simulink library "beamform"  (Simulink 7.0)
libraries: xbsIndex_r4 x216, beamform x73
(part 1 of 2)
settings Model: Creator=Administrator  LastModifiedBy=Administrator

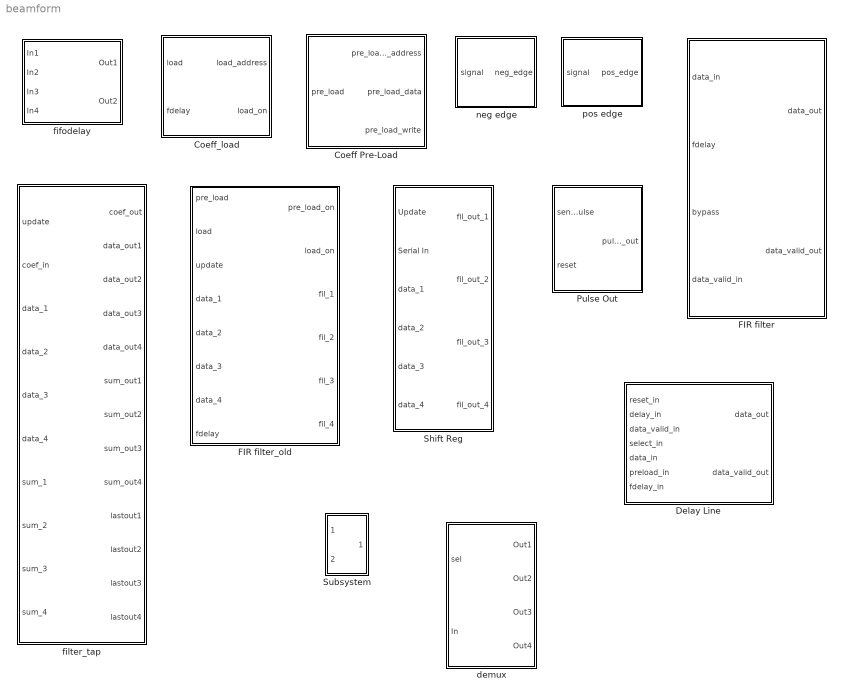
== system beamform ==
  Coeff Pre-Load : Subsystem  mask{N=20, T=10, bin_pnt=6, file='cfile.mat'}
      mask prompts: N "No of Filters"; T "No of Taps"; bin_pnt "Binary Point"; file "Coefficients File"
      mask init:
      | load(file)
  Coeff_load : Subsystem  mask{nfilters=10, ntaps=20}
      mask prompts: nfilters "Number of FD filters"; ntaps "Number of Taps per filter"
      mask init:
      | coef_load;
  Delay Line : Subsystem
  FIR filter : Subsystem
  FIR filter_old : Subsystem  mask{ntaps=4, nfilters=4, cfile=test.mat, bin_pnt=6}
      mask prompts: ntaps "No of Taps"; nfilters "No of Filters"; cfile "Coefficients"; bin_pnt "Binary Point"
      mask init:
      | load(cfile);
  Pulse Out : Subsystem
  Shift Reg : Subsystem  mask{n=20, bin_point=6}
      mask prompts: n "No of taps"; bin_point "Binary Point"
      mask init:
      | shift_reg;
  Subsystem : Subsystem
  demux : Subsystem  mask{n_bits=20}
  fifodelay : Subsystem  mask{depth=1}
      mask init:
      | drawfifo;
      mask Display:
      | port_label('input',1,'reset');
      | port_label('input',2,'data_in');
      | port_label('input',3,'delay');
      | port_label('input',4,'data_valid');
      | port_label('output',1,'data_out');
      | port_label('output',2,'data_valid');
  filter_tap : Subsystem  mask{n_bits=8, bnpnt=6, mux_latency=0, add_latency=2, mult_latency=3, qn_bits=18, qbnpnt=16}
      mask prompts: n_bits "Coefficient bit width"; bnpnt "Coeff & Data Binary Point"; mux_latency "Multiplexer Latency"; add_latency "Add Latency"; mult_latency "Multiplier Latency"; qn_bits "Quiscent Bitwdith"; qbnpnt "Quiscent Binary Point"
  neg edge : Subsystem  mask{add_latency=1}
  pos edge : Subsystem  mask{add_latency=1}

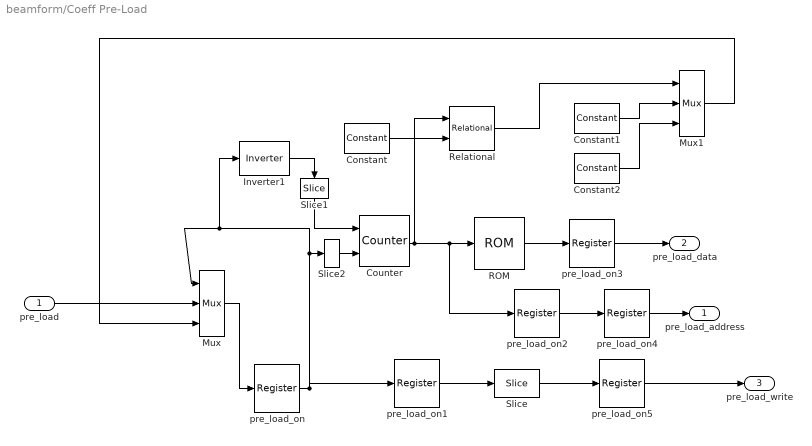
== system beamform/Coeff Pre-Load ==
  pre_load : Inport  OutDataType=sfix(16)  OutScaling=2^0
  Constant : xbsIndex_r4/Constant  arith_type=Unsigned  const=N*T-1  n_bits=ceil(log2(N*T-1))  bin_pt=0  explicit_period=on  period=1  equ=P=C  opselect=C  inp2=PCIN>>17  opr=+  inp1=P  carry=CIN  dbl_ovrd=off  block_type=constant
  Constant1 : xbsIndex_r4/Constant  arith_type=Unsigned  const=1  n_bits=1  bin_pt=0  explicit_period=on  period=1  equ=P=C  opselect=C  inp2=PCIN>>17  opr=+  inp1=P  carry=CIN  dbl_ovrd=off  block_type=constant
  Constant2 : xbsIndex_r4/Constant  arith_type=Unsigned  const=0  n_bits=1  bin_pt=0  explicit_period=on  period=1  equ=P=C  opselect=C  inp2=PCIN>>17  opr=+  inp1=P  carry=CIN  dbl_ovrd=off  block_type=constant
  Counter : xbsIndex_r4/Counter  cnt_type=Count Limited  cnt_to=N*T-1  operation=Up  start_count=0  cnt_by_val=1  arith_type=Unsigned  n_bits=ceil(log2(N*T))  bin_pt=0  load_pin=off  rst=on  en=on  explicit_period=off  period=1  dbl_ovrd=off  use_behavioral_HDL=off  use_rpm=on  implementation=Fabric  block_type=counter
      settings: xl_area=[0, 0, 0, 0, 0, 0, 0]
  Inverter1 : xbsIndex_r4/Inverter  en=off  latency=0  dbl_ovrd=off  block_type=inv
      settings: xl_area=[0, 0, 0, 0, 0, 0, 0]
  Mux : xbsIndex_r4/Mux  inputs=2  en=off  latency=0  precision=Full  arith_type=Unsigned  n_bits=1  bin_pt=0  quantization=Truncate  overflow=Wrap  dbl_ovrd=off  block_type=mux
      settings: xl_area=[0, 0, 0, 0, 0, 0, 0]
  Mux1 : xbsIndex_r4/Mux  inputs=2  en=off  latency=0  precision=Full  arith_type=Unsigned  n_bits=1  bin_pt=0  quantization=Truncate  overflow=Wrap  dbl_ovrd=off  block_type=mux
      settings: xl_area=[0, 0, 0, 0, 0, 0, 0]
  ROM : xbsIndex_r4/ROM  depth=N*T  initVector=A  distributed_mem=Block RAM  rst=off  init_reg=0  en=off  latency=1  arith_type="Signed  (2's comp)"  n_bits=18  bin_pt=16  dbl_ovrd=off  optimize=Area  use_rpm=off  block_type=sprom
      settings: xl_area=[0, 0, 0, 0, 0, 0, 0]  block_version=10.1.3
  Relational : xbsIndex_r4/Relational  mode=a>=b  en=off  latency=1  dbl_ovrd=off  block_type=relational
      settings: xl_area=[0, 0, 0, 0, 0, 0, 0]  block_version=10.1.3
  Slice : xbsIndex_r4/Slice  nbits=1  boolean_output=on  mode=Upper Bit Location + Width  bit1=0  base1=MSB of Input  bit0=0  base0=LSB of Input  dbl_ovrd=off  block_type=slice
      settings: infoedit="Extracts a given range of bits from each input sample and presents it at the output.  The output type is ordinarily unsigned with binary point at zero, but can be Boolean when the slice is one bit wide.<P><P>Hardware notes: In hardware this block costs nothing."  block_version=10.1.3
  Slice1 : xbsIndex_r4/Slice  Orientation=down  nbits=1  boolean_output=on  mode=Upper Bit Location + Width  bit1=0  base1=MSB of Input  bit0=0  base0=LSB of Input  dbl_ovrd=off  block_type=slice
      settings: infoedit="Extracts a given range of bits from each input sample and presents it at the output.  The output type is ordinarily unsigned with binary point at zero, but can be Boolean when the slice is one bit wide.<P><P>Hardware notes: In hardware this block costs nothing."  block_version=10.1.3
  Slice2 : xbsIndex_r4/Slice  nbits=1  boolean_output=on  mode=Upper Bit Location + Width  bit1=0  base1=MSB of Input  bit0=0  base0=LSB of Input  dbl_ovrd=off  block_type=slice
      settings: infoedit="Extracts a given range of bits from each input sample and presents it at the output.  The output type is ordinarily unsigned with binary point at zero, but can be Boolean when the slice is one bit wide.<P><P>Hardware notes: In hardware this block costs nothing."  block_version=10.1.3
  pre_load_on{,1..5} (6 alike) : xbsIndex_r4/Register  init=0  rst=off  en=off  dbl_ovrd=off  block_type=register
      settings: xl_area=[0, 0, 0, 0, 0, 0, 0]
  pre_load_address : Outport  OutDataType=sfix(16)  OutScaling=2^0
  pre_load_data : Outport  Port=2  OutDataType=sfix(16)  OutScaling=2^0
  pre_load_write : Outport  Port=3  OutDataType=sfix(16)  OutScaling=2^0
  wires:
  pre_load_on5/1 -> pre_load_write/1
  pre_load_on4/1 -> pre_load_address/1
  pre_load_on3/1 -> pre_load_data/1
  Slice2/1 -> Counter/2
  Slice1/1 -> Counter/1
  Mux1/1 -> Mux/3
  Constant2/1 -> Mux1/3
  Constant1/1 -> Mux1/2
  Relational/1 -> Mux1/1
  Slice/1 -> pre_load_on5/1
  Counter/1 -> pre_load_on2/1, ROM/1, Relational/1
  ROM/1 -> pre_load_on3/1
  Constant/1 -> Relational/2
  pre_load_on/1 -> pre_load_on1/1, Slice2/1, Mux/1, Inverter1/1
  Inverter1/1 -> Slice1/1
  Mux/1 -> pre_load_on/1
  pre_load/1 -> Mux/2
  pre_load_on1/1 -> Slice/1
  pre_load_on2/1 -> pre_load_on4/1

== system beamform/Coeff_load ==
  load : Inport  OutDataType=sfix(16)  OutScaling=2^0
  fdelay : Inport  Port=2  OutDataType=sfix(16)  OutScaling=2^0
  AddSub : xbsIndex_r4/AddSub  mode=Addition  use_carryin=off  use_carryout=off  en=off  latency=1  precision=User Defined  arith_type=Unsigned  n_bits=8  bin_pt=0  quantization=Truncate  overflow=Wrap  dbl_ovrd=off  use_behavioral_HDL=on  pipelined=off  use_rpm=on  hw_selection=Fabric  block_type=addsub
      settings: xl_area=[0, 0, 0, 0, 0, 0, 0]  block_version=10.1.3
  Constant : xbsIndex_r4/Constant  arith_type=Unsigned  const=19  n_bits=5  bin_pt=0  explicit_period=on  period=1  equ=P=C  opselect=C  inp2=PCIN>>17  opr=+  inp1=P  carry=CIN  dbl_ovrd=off  block_type=constant
  Counter : xbsIndex_r4/Counter  cnt_type=Count Limited  cnt_to=19  operation=Up  start_count=0  cnt_by_val=1  arith_type=Unsigned  n_bits=5  bin_pt=0  load_pin=off  rst=on  en=on  explicit_period=off  period=1  dbl_ovrd=off  use_behavioral_HDL=off  use_rpm=on  implementation=Fabric  block_type=counter
      settings: xl_area=[0, 0, 0, 0, 0, 0, 0]
  Inverter : xbsIndex_r4/Inverter  Orientation=left  en=off  latency=0  dbl_ovrd=off  block_type=inv
      settings: xl_area=[0, 0, 0, 0, 0, 0, 0]
  Inverter1 : xbsIndex_r4/Inverter  Orientation=up  en=off  latency=0  dbl_ovrd=off  block_type=inv
      settings: xl_area=[0, 0, 0, 0, 0, 0, 0]
  Mux : xbsIndex_r4/Mux  inputs=2  en=off  latency=0  precision=Full  arith_type="Signed  (2's comp)"  n_bits=8  bin_pt=2  quantization=Truncate  overflow=Wrap  dbl_ovrd=off  block_type=mux
      settings: xl_area=[0, 0, 0, 0, 0, 0, 0]
  Mux1 : xbsIndex_r4/Mux  inputs=10  en=off  latency=1  precision=Full  arith_type="Signed  (2's comp)"  n_bits=8  bin_pt=2  quantization=Truncate  overflow=Wrap  dbl_ovrd=off  block_type=mux
      settings: xl_area=[0, 0, 0, 0, 0, 0, 0]
  Relational : xbsIndex_r4/Relational  mode=a>=b  en=off  latency=1  dbl_ovrd=off  block_type=relational
      settings: xl_area=[0, 0, 0, 0, 0, 0, 0]  block_version=10.1.3
  load_on1 : xbsIndex_r4/Register  init=0  rst=off  en=off  dbl_ovrd=off  block_type=register
      settings: xl_area=[0, 0, 0, 0, 0, 0, 0]
  load_on2 : xbsIndex_r4/Register  init=0  rst=off  en=off  dbl_ovrd=off  block_type=register
      settings: xl_area=[0, 0, 0, 0, 0, 0, 0]
  load_on3 : xbsIndex_r4/Register  init=0  rst=off  en=off  dbl_ovrd=off  block_type=register
      settings: xl_area=[0, 0, 0, 0, 0, 0, 0]
  load_address : Outport  OutDataType=sfix(16)  OutScaling=2^0
  load_on : Outport  Port=2  OutDataType=sfix(16)  OutScaling=2^0
  wires:
  load_on3/1 -> load_on/1
  load_on2/1 -> load_on3/1
  Counter/1 -> Relational/1, AddSub/1
  Constant/1 -> Relational/2
  Relational/1 -> Inverter/1
  load_on1/1 -> load_on2/1, Counter/2, Mux/1, Inverter1/1
  Inverter/1 -> Mux/3
  Mux/1 -> load_on1/1
  load/1 -> Mux/2
  Inverter1/1 -> Counter/1
  fdelay/1 -> Mux1/1
  Mux1/1 -> AddSub/2
  AddSub/1 -> load_address/1

== system beamform/Delay Line ==
  reset_in : Inport  OutDataType=sfix(16)  OutScaling=2^0
  delay_in : Inport  Port=2  OutDataType=sfix(16)  OutScaling=2^0
  data_valid_in : Inport  Port=3  OutDataType=sfix(16)  OutScaling=2^0
  select_in : Inport  Port=4  OutDataType=sfix(16)  OutScaling=2^0
  data_in : Inport  Port=5  OutDataType=sfix(16)  OutScaling=2^0
  preload_in : Inport  Port=6  OutDataType=sfix(16)  OutScaling=2^0
  fdelay_in : Inport  Port=7  OutDataType=sfix(16)  OutScaling=2^0
  Concat : xbsIndex_r4/Concat  num_inputs=4  dbl_ovrd=off  block_type=concat
      settings: block_version=10.1.3
  FIR filter : Subsystem  AncestorBlock=beamform/FIR filter
  Fifo : Subsystem
  Mux : Subsystem
  Slice : xbsIndex_r4/Slice  nbits=8  boolean_output=off  mode=Two Bit Locations  bit1=31  base1=LSB of Input  bit0=0  base0=LSB of Input  dbl_ovrd=off  block_type=slice
      settings: infoedit="Extracts a given range of bits from each input sample and presents it at the output.  The output type is ordinarily unsigned with binary point at zero, but can be Boolean when the slice is one bit wide.<P><P>Hardware notes: In hardware this block costs nothing."  block_version=10.1.3
  Slice1 : xbsIndex_r4/Slice  nbits=8  boolean_output=off  mode=Two Bit Locations  bit1=23  base1=LSB of Input  bit0=16  base0=LSB of Input  dbl_ovrd=off  block_type=slice
      settings: infoedit="Extracts a given range of bits from each input sample and presents it at the output.  The output type is ordinarily unsigned with binary point at zero, but can be Boolean when the slice is one bit wide.<P><P>Hardware notes: In hardware this block costs nothing."  block_version=10.1.3
  Slice2 : xbsIndex_r4/Slice  nbits=8  boolean_output=off  mode=Two Bit Locations  bit1=15  base1=LSB of Input  bit0=8  base0=LSB of Input  dbl_ovrd=off  block_type=slice
      settings: infoedit="Extracts a given range of bits from each input sample and presents it at the output.  The output type is ordinarily unsigned with binary point at zero, but can be Boolean when the slice is one bit wide.<P><P>Hardware notes: In hardware this block costs nothing."  block_version=10.1.3
  Slice3 : xbsIndex_r4/Slice  nbits=8  boolean_output=off  mode=Two Bit Locations  bit1=7  base1=LSB of Input  bit0=0  base0=LSB of Input  dbl_ovrd=off  block_type=slice
      settings: infoedit="Extracts a given range of bits from each input sample and presents it at the output.  The output type is ordinarily unsigned with binary point at zero, but can be Boolean when the slice is one bit wide.<P><P>Hardware notes: In hardware this block costs nothing."  block_version=10.1.3
  data_out : Outport  OutDataType=sfix(16)  OutScaling=2^0
  data_valid_out : Outport  Port=2  OutDataType=sfix(16)  OutScaling=2^0
  wires:
  Fifo/1(data_out) -> Mux/1(data_in)
  Fifo/2(data_valid_out) -> Mux/2(data_valid_in)
  reset_in/1 -> Fifo/1(reset_in), Mux/3(reset_in)
  delay_in/1 -> Fifo/2(delay_in)
  data_valid_in/1 -> Fifo/3(data_valid_in)
  Mux/2(data_valid_out) -> data_valid_out/1
  select_in/1 -> Mux/4(select)
  data_in/1 -> Fifo/4(data_in)
  Mux/1(data_out) -> Slice/1, Slice1/1, Slice2/1, Slice3/1
  Slice/1 -> FIR filter/2(data_1)
  Slice1/1 -> FIR filter/3(data_2)
  Slice2/1 -> FIR filter/4(data_3)
  Slice3/1 -> FIR filter/5(data_4)
  FIR filter/1(fil_1) -> Concat/1
  FIR filter/2(fil_2) -> Concat/2
  FIR filter/3(fil_3) -> Concat/3
  FIR filter/4(fil_4) -> Concat/4
  Concat/1 -> data_out/1
  preload_in/1 -> FIR filter/1(pre_load)
  fdelay_in/1 -> FIR filter/6(fdelay)

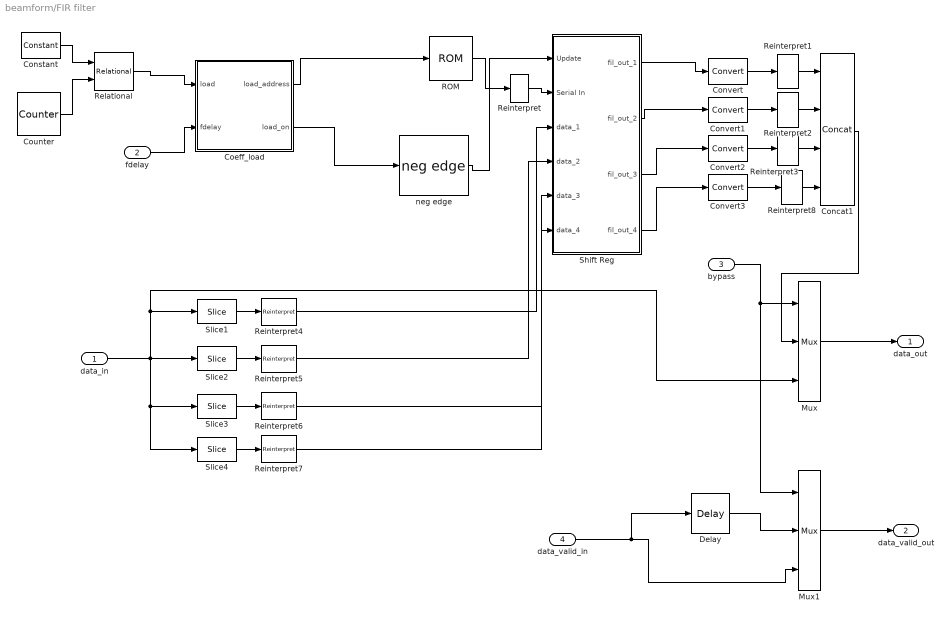
== system beamform/FIR filter ==
  data_in : Inport  OutDataType=sfix(16)  OutScaling=2^0
  fdelay : Inport  Port=2  OutDataType=sfix(16)  OutScaling=2^0
  bypass : Inport  Port=3  OutDataType=sfix(16)  OutScaling=2^0
  data_valid_in : Inport  Port=4  OutDataType=sfix(16)  OutScaling=2^0
  Coeff_load : Subsystem  AncestorBlock=beamform/Coeff_load  mask{nfilters=10, ntaps=10}
      mask prompts: nfilters "Number of FD filters"; ntaps "Number of Taps per filter"
      mask init:
      | coef_load;
  Concat1 : xbsIndex_r4/Concat  num_inputs=4  dbl_ovrd=off  block_type=concat
      settings: block_version=10.1.3
  Constant : xbsIndex_r4/Constant  arith_type=Unsigned  const=0  n_bits=11  bin_pt=0  explicit_period=on  period=1  equ=P=C  opselect=C  inp2=PCIN>>17  opr=+  inp1=P  carry=CIN  dbl_ovrd=off  block_type=constant
  Convert{,1..3} (4 alike) : xbsIndex_r4/Convert  arith_type="Signed  (2's comp)"  n_bits=8  bin_pt=6  quantization=Truncate  overflow=Wrap  latency=0  dbl_ovrd=off  pipeline=off  block_type=convert
      settings: xl_area=[0, 0, 0, 0, 0, 0, 0]  block_version=10.1.3
  Counter : xbsIndex_r4/Counter  cnt_type=Free Running  cnt_to=Inf  operation=Up  start_count=0  cnt_by_val=1  arith_type=Unsigned  n_bits=11  bin_pt=0  load_pin=off  rst=off  en=off  explicit_period=off  period=1  dbl_ovrd=off  use_behavioral_HDL=off  use_rpm=on  implementation=Fabric  block_type=counter
      settings: xl_area=[0, 0, 0, 0, 0, 0, 0]
  Delay : xbsIndex_r4/Delay  en=off  latency=10*6  dbl_ovrd=off  reg_retiming=off  block_type=delay
      settings: xl_area=[0, 0, 0, 0, 0, 0, 0]
  Mux : xbsIndex_r4/Mux  inputs=2  en=off  latency=1  precision=Full  arith_type="Signed  (2's comp)"  n_bits=8  bin_pt=2  quantization=Truncate  overflow=Wrap  dbl_ovrd=off  block_type=mux
      settings: xl_area=[0, 0, 0, 0, 0, 0, 0]
  Mux1 : xbsIndex_r4/Mux  inputs=2  en=off  latency=1  precision=Full  arith_type="Signed  (2's comp)"  n_bits=8  bin_pt=2  quantization=Truncate  overflow=Wrap  dbl_ovrd=off  block_type=mux
      settings: xl_area=[0, 0, 0, 0, 0, 0, 0]
  ROM : xbsIndex_r4/ROM  depth=100  initVector=A  distributed_mem=Block RAM  rst=off  init_reg=0  en=off  latency=1  arith_type="Signed  (2's comp)"  n_bits=18  bin_pt=16  dbl_ovrd=off  optimize=Area  use_rpm=off  block_type=sprom
      settings: xl_area=[0, 0, 0, 0, 0, 0, 0]  block_version=10.1.3
  Reinterpret : xbsIndex_r4/Reinterpret  force_arith_type=on  arith_type="Signed  (2's comp)"  force_bin_pt=on  bin_pt=16  block_type=reinterpret
      settings: infoedit="Changes signal type without altering the binary representation.   You can changed the signal between signed and unsigned, and relocate the binary point.<P><P>Hardware notes: In hardware this block costs nothing.<P><P>Example:  Suppose the input is 6 bits wide, signed, with 2 fractional bits, and the output is forced to unsigned with 0 fractional bits.  Then an input of -2.0 (1110.00 in binary 2's complement) becomes an output of 56 (111000 in binary)."  block_version=10.1.3
  Reinterpret{1..3,8} (4 alike) : xbsIndex_r4/Reinterpret  force_arith_type=on  arith_type=Unsigned  force_bin_pt=on  bin_pt=0  block_type=reinterpret
      settings: infoedit="Changes signal type without altering the binary representation.   You can changed the signal between signed and unsigned, and relocate the binary point.<P><P>Hardware notes: In hardware this block costs nothing.<P><P>Example:  Suppose the input is 6 bits wide, signed, with 2 fractional bits, and the output is forced to unsigned with 0 fractional bits.  Then an input of -2.0 (1110.00 in binary 2's complement) becomes an output of 56 (111000 in binary)."  block_version=10.1.3
  Reinterpret{4..7} (4 alike) : xbsIndex_r4/Reinterpret  force_arith_type=on  arith_type="Signed  (2's comp)"  force_bin_pt=on  bin_pt=6  block_type=reinterpret
      settings: infoedit="Changes signal type without altering the binary representation.   You can changed the signal between signed and unsigned, and relocate the binary point.<P><P>Hardware notes: In hardware this block costs nothing.<P><P>Example:  Suppose the input is 6 bits wide, signed, with 2 fractional bits, and the output is forced to unsigned with 0 fractional bits.  Then an input of -2.0 (1110.00 in binary 2's complement) becomes an output of 56 (111000 in binary)."  block_version=10.1.3
  Relational : xbsIndex_r4/Relational  mode=a=b  en=off  latency=1  dbl_ovrd=off  block_type=relational
      settings: xl_area=[0, 0, 0, 0, 0, 0, 0]  block_version=10.1.3
  Shift Reg : Subsystem  AncestorBlock=beamform/Shift Reg  mask{n=10, bin_point=6}
      mask prompts: n "No of taps"; bin_point "Binary Point"
      mask init:
      | shift_reg;
  Slice1 : xbsIndex_r4/Slice  nbits=8  boolean_output=off  mode=Two Bit Locations  bit1=31  base1=LSB of Input  bit0=24  base0=LSB of Input  dbl_ovrd=off  block_type=slice
      settings: infoedit="Extracts a given range of bits from each input sample and presents it at the output.  The output type is ordinarily unsigned with binary point at zero, but can be Boolean when the slice is one bit wide.<P><P>Hardware notes: In hardware this block costs nothing."  block_version=10.1.3
  Slice2 : xbsIndex_r4/Slice  nbits=8  boolean_output=off  mode=Two Bit Locations  bit1=23  base1=LSB of Input  bit0=16  base0=LSB of Input  dbl_ovrd=off  block_type=slice
      settings: infoedit="Extracts a given range of bits from each input sample and presents it at the output.  The output type is ordinarily unsigned with binary point at zero, but can be Boolean when the slice is one bit wide.<P><P>Hardware notes: In hardware this block costs nothing."  block_version=10.1.3
  Slice3 : xbsIndex_r4/Slice  nbits=8  boolean_output=off  mode=Two Bit Locations  bit1=15  base1=LSB of Input  bit0=8  base0=LSB of Input  dbl_ovrd=off  block_type=slice
      settings: infoedit="Extracts a given range of bits from each input sample and presents it at the output.  The output type is ordinarily unsigned with binary point at zero, but can be Boolean when the slice is one bit wide.<P><P>Hardware notes: In hardware this block costs nothing."  block_version=10.1.3
  Slice4 : xbsIndex_r4/Slice  nbits=8  boolean_output=off  mode=Two Bit Locations  bit1=7  base1=LSB of Input  bit0=0  base0=LSB of Input  dbl_ovrd=off  block_type=slice
      settings: infoedit="Extracts a given range of bits from each input sample and presents it at the output.  The output type is ordinarily unsigned with binary point at zero, but can be Boolean when the slice is one bit wide.<P><P>Hardware notes: In hardware this block costs nothing."  block_version=10.1.3
  neg edge : beamform/neg edge  SystemSampleTime=-1  add_latency=1
  data_out : Outport  OutDataType=sfix(16)  OutScaling=2^0
  data_valid_out : Outport  Port=2  OutDataType=sfix(16)  OutScaling=2^0
  wires:
  Counter/1 -> Relational/2
  Constant/1 -> Relational/1
  Mux1/1 -> data_valid_out/1
  Delay/1 -> Mux1/2
  data_valid_in/1 -> Delay/1, Mux1/3
  Reinterpret8/1 -> Concat1/4
  Reinterpret3/1 -> Concat1/3
  Reinterpret2/1 -> Concat1/2
  Reinterpret1/1 -> Concat1/1
  Concat1/1 -> Mux/2
  bypass/1 -> Mux1/1, Mux/1
  Mux/1 -> data_out/1
  Convert3/1 -> Reinterpret8/1
  Convert2/1 -> Reinterpret3/1
  Convert1/1 -> Reinterpret2/1
  Convert/1 -> Reinterpret1/1
  Shift Reg/4(fil_out_4) -> Convert3/1
  Shift Reg/3(fil_out_3) -> Convert2/1
  Shift Reg/2(fil_out_2) -> Convert1/1
  Shift Reg/1(fil_out_1) -> Convert/1
  Reinterpret7/1 -> Shift Reg/6(data_4)
  Reinterpret6/1 -> Shift Reg/5(data_3)
  Reinterpret5/1 -> Shift Reg/4(data_2)
  Reinterpret4/1 -> Shift Reg/3(data_1)
  data_in/1 -> Mux/3, Slice1/1, Slice4/1, Slice3/1, Slice2/1
  Slice4/1 -> Reinterpret7/1
  Slice3/1 -> Reinterpret6/1
  Slice2/1 -> Reinterpret5/1
  Slice1/1 -> Reinterpret4/1
  fdelay/1 -> Coeff_load/2(fdelay)
  Coeff_load/2(load_on) -> neg edge/1
  ROM/1 -> Reinterpret/1
  Coeff_load/1(load_address) -> ROM/1
  Relational/1 -> Coeff_load/1(load)
  neg edge/1 -> Shift Reg/1(Update)
  Reinterpret/1 -> Shift Reg/2(Serial In)

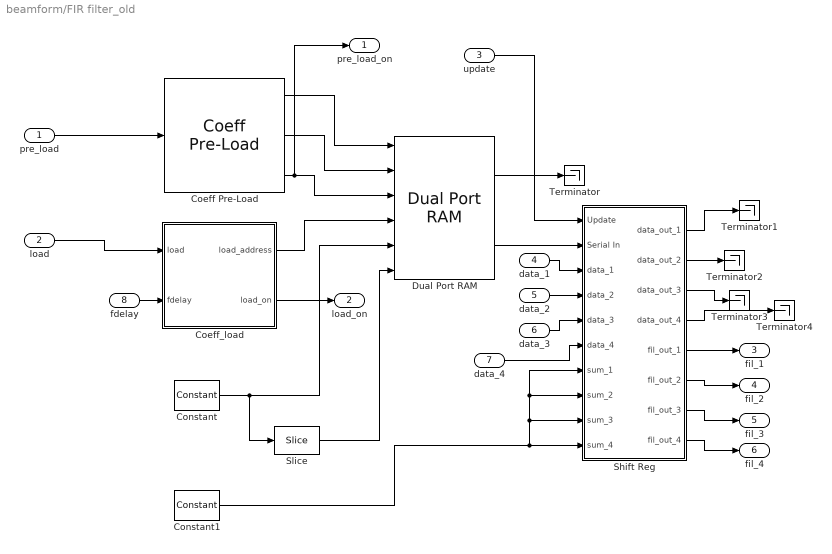
== system beamform/FIR filter_old ==
  pre_load : Inport  OutDataType=sfix(16)  OutScaling=2^0
  load : Inport  Port=2  OutDataType=sfix(16)  OutScaling=2^0
  update : Inport  Port=3  OutDataType=sfix(16)  OutScaling=2^0
  data_1 : Inport  Port=4  OutDataType=sfix(16)  OutScaling=2^0
  data_2 : Inport  Port=5  OutDataType=sfix(16)  OutScaling=2^0
  data_3 : Inport  Port=6  OutDataType=sfix(16)  OutScaling=2^0
  data_4 : Inport  Port=7  OutDataType=sfix(16)  OutScaling=2^0
  fdelay : Inport  Port=8  OutDataType=sfix(16)  OutScaling=2^0
  Coeff Pre-Load : beamform/Coeff Pre-Load  SystemSampleTime=-1  N=nfilters  T=ntaps  bin_pnt=bin_pnt  file=cfile
  Coeff_load : Subsystem  AncestorBlock=beamform/Coeff_load  mask{nfilters=nfilters, ntaps=ntaps}
      mask prompts: nfilters "Number of FD filters"; ntaps "Number of Taps per filter"
      mask init:
      | coef_load;
  Constant : xbsIndex_r4/Constant  arith_type=Unsigned  const=0  n_bits=8  bin_pt=0  explicit_period=off  period=1  equ=P=C  opselect=C  inp2=PCIN>>17  opr=+  inp1=P  carry=CIN  dbl_ovrd=off  block_type=constant
  Constant1 : xbsIndex_r4/Constant  arith_type=Unsigned  const=0  n_bits=18  bin_pt=6  explicit_period=off  period=1  equ=P=C  opselect=C  inp2=PCIN>>17  opr=+  inp1=P  carry=CIN  dbl_ovrd=off  block_type=constant
  Dual Port RAM : xbsIndex_r4/Dual Port RAM  depth=ntaps*nfilters  initVector=sin(pi*(0:15)/16)  distributed_mem=Block RAM  init_a=0  init_b=0  rst_a=off  rst_b=off  en_a=off  en_b=off  latency=1  write_mode_A=Read Before Write  write_mode_B=Read Before Write  dbl_ovrd=off  optimize=Area  use_rpm=off  block_type=dpram
      settings: xl_area=[0, 0, 0, 0, 0, 0, 0]  block_version=10.1.3
  Shift Reg : Subsystem  AncestorBlock=beamform/Shift Reg  mask{n=ntaps, bin_point=bin_pnt}
      mask prompts: n "No of taps"; bin_point "Binary Point"
      mask init:
      | shift_reg;
  Slice : xbsIndex_r4/Slice  nbits=1  boolean_output=off  mode=Lower Bit Location + Width  bit1=0  base1=MSB of Input  bit0=0  base0=LSB of Input  dbl_ovrd=off  block_type=slice
      settings: infoedit="Extracts a given range of bits from each input sample and presents it at the output.  The output type is ordinarily unsigned with binary point at zero, but can be Boolean when the slice is one bit wide.<P><P>Hardware notes: In hardware this block costs nothing."  block_version=10.1.3
  Terminator{,1..4} (5 alike) : Terminator
  pre_load_on : Outport  OutDataType=sfix(16)  OutScaling=2^0
  load_on : Outport  Port=2  OutDataType=sfix(16)  OutScaling=2^0
  fil_1 : Outport  Port=3  OutDataType=sfix(16)  OutScaling=2^0
  fil_2 : Outport  Port=4  OutDataType=sfix(16)  OutScaling=2^0
  fil_3 : Outport  Port=5  OutDataType=sfix(16)  OutScaling=2^0
  fil_4 : Outport  Port=6  OutDataType=sfix(16)  OutScaling=2^0
  wires:
  Coeff Pre-Load/1 -> Dual Port RAM/1
  Coeff Pre-Load/2 -> Dual Port RAM/2
  Coeff Pre-Load/3 -> Dual Port RAM/3, pre_load_on/1
  Coeff_load/1(load_address) -> Dual Port RAM/4
  Constant/1 -> Dual Port RAM/5, Slice/1
  Slice/1 -> Dual Port RAM/6
  Dual Port RAM/2 -> Shift Reg/2(Serial In)
  Constant1/1 -> Shift Reg/10(sum_4), Shift Reg/9(sum_3), Shift Reg/8(sum_2), Shift Reg/7(sum_1)
  pre_load/1 -> Coeff Pre-Load/1
  load/1 -> Coeff_load/1(load)
  update/1 -> Shift Reg/1(Update)
  data_4/1 -> Shift Reg/6(data_4)
  data_3/1 -> Shift Reg/5(data_3)
  data_2/1 -> Shift Reg/4(data_2)
  data_1/1 -> Shift Reg/3(data_1)
  Shift Reg/5(fil_out_1) -> fil_1/1
  Shift Reg/6(fil_out_2) -> fil_2/1
  Shift Reg/7(fil_out_3) -> fil_3/1
  Shift Reg/8(fil_out_4) -> fil_4/1
  Coeff_load/2(load_on) -> load_on/1
  Dual Port RAM/1 -> Terminator/1
  Shift Reg/3(data_out_3) -> Terminator3/1
  fdelay/1 -> Coeff_load/2(fdelay)
  Shift Reg/4(data_out_4) -> Terminator4/1
  Shift Reg/1(data_out_1) -> Terminator1/1
  Shift Reg/2(data_out_2) -> Terminator2/1

== system beamform/Pulse Out ==
  send_pulse : Inport  OutDataType=sfix(16)  OutScaling=2^0
  reset : Inport  Port=2  OutDataType=sfix(16)  OutScaling=2^0
  Inverter : xbsIndex_r4/Inverter  en=off  latency=0  dbl_ovrd=off  block_type=inv
      settings: xl_area=[0, 0, 0, 0, 0, 0, 0]
  Logical : xbsIndex_r4/Logical  logical_function=AND  inputs=2  en=off  latency=0  precision=Full  arith_type=Unsigned  n_bits=8  bin_pt=2  align_bp=on  dbl_ovrd=off  block_type=logical
      settings: xl_area=[0, 0, 0, 0, 0, 0, 0]
  Logical1 : xbsIndex_r4/Logical  logical_function=AND  inputs=2  en=off  latency=0  precision=User Defined  arith_type=Unsigned  n_bits=1  bin_pt=0  align_bp=on  dbl_ovrd=off  block_type=logical
      settings: xl_area=[0, 0, 0, 0, 0, 0, 0]
  Mux : xbsIndex_r4/Mux  inputs=2  en=off  latency=0  precision=Full  arith_type="Signed  (2's comp)"  n_bits=8  bin_pt=2  quantization=Truncate  overflow=Wrap  dbl_ovrd=off  block_type=mux
      settings: xl_area=[0, 0, 0, 0, 0, 0, 0]
  pulse_done : xbsIndex_r4/Register  init=0  rst=on  en=off  dbl_ovrd=off  block_type=register
      settings: xl_area=[0, 0, 0, 0, 0, 0, 0]
  pulse_out : Outport  OutDataType=sfix(16)  OutScaling=2^0
  wires:
  Mux/1 -> pulse_done/1
  pulse_done/1 -> Logical/2, Inverter/1
  send_pulse/1 -> Logical/1, Logical1/1, Mux/3
  Logical/1 -> Mux/1
  Logical1/1 -> pulse_out/1, Mux/2
  Inverter/1 -> Logical1/2
  reset/1 -> pulse_done/2

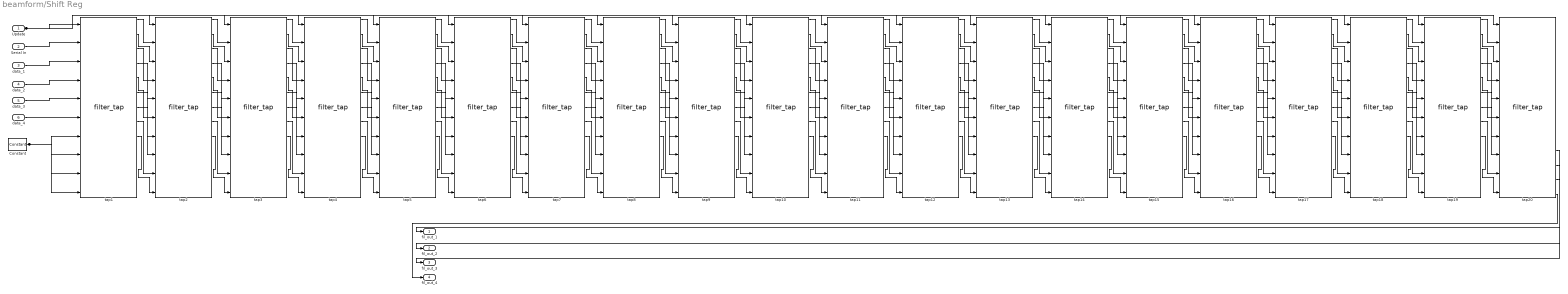
== system beamform/Shift Reg ==
  Update : Inport  OutDataType=sfix(16)  OutScaling=2^0
  Serial In : Inport  Port=2  OutDataType=sfix(16)  OutScaling=2^0
  data_1 : Inport  Port=3  OutDataType=sfix(16)  OutScaling=2^0
  data_2 : Inport  Port=4  OutDataType=sfix(16)  OutScaling=2^0
  data_3 : Inport  Port=5  OutDataType=sfix(16)  OutScaling=2^0
  data_4 : Inport  Port=6  OutDataType=sfix(16)  OutScaling=2^0
  Constant : xbsIndex_r4/Constant  arith_type=Signed (2's comp)  const=0  n_bits=18  bin_pt=6  explicit_period=on  period=1  equ=P=C  opselect=C  inp2=PCIN>>17  opr=+  inp1=P  carry=CIN  dbl_ovrd=off  block_type=constant
  tap{1..20} (20 alike) : beamform/filter_tap  SystemSampleTime=-1  n_bits=8  bnpnt=6  mux_latency=0  add_latency=2  mult_latency=3  qn_bits=18  qbnpnt=16
  fil_out_1 : Outport  OutDataType=sfix(16)  OutScaling=2^0
  fil_out_2 : Outport  Port=2  OutDataType=sfix(16)  OutScaling=2^0
  fil_out_3 : Outport  Port=3  OutDataType=sfix(16)  OutScaling=2^0
  fil_out_4 : Outport  Port=4  OutDataType=sfix(16)  OutScaling=2^0
  wires:
  Constant/1 -> tap1/7, tap1/8, tap1/9, tap1/10
  Update/1 -> tap1/1, tap2/1, tap3/1, tap4/1, tap5/1, tap6/1, tap7/1, tap8/1, tap9/1, tap10/1, tap11/1, tap12/1, tap13/1, tap14/1, tap15/1, tap16/1, tap17/1, tap18/1, tap19/1, tap20/1
  Serial In/1 -> tap1/2
  data_1/1 -> tap1/3
  data_2/1 -> tap1/4
  data_3/1 -> tap1/5
  data_4/1 -> tap1/6
  tap1/1 -> tap2/2
  tap1/2 -> tap2/3
  tap1/3 -> tap2/4
  tap1/4 -> tap2/5
  tap1/5 -> tap2/6
  tap1/6 -> tap2/7
  tap1/7 -> tap2/8
  tap1/8 -> tap2/9
  tap1/9 -> tap2/10
  tap2/1 -> tap3/2
  tap2/2 -> tap3/3
  tap2/3 -> tap3/4
  tap2/4 -> tap3/5
  tap2/5 -> tap3/6
  tap2/6 -> tap3/7
  tap2/7 -> tap3/8
  tap2/8 -> tap3/9
  tap2/9 -> tap3/10
  tap3/1 -> tap4/2
  tap3/2 -> tap4/3
  tap3/3 -> tap4/4
  tap3/4 -> tap4/5
  tap3/5 -> tap4/6
  tap3/6 -> tap4/7
  tap3/7 -> tap4/8
  tap3/8 -> tap4/9
  tap3/9 -> tap4/10
  tap4/1 -> tap5/2
  tap4/2 -> tap5/3
  tap4/3 -> tap5/4
  tap4/4 -> tap5/5
  tap4/5 -> tap5/6
  tap4/6 -> tap5/7
  tap4/7 -> tap5/8
  tap4/8 -> tap5/9
  tap4/9 -> tap5/10
  tap5/1 -> tap6/2
  tap5/2 -> tap6/3
  tap5/3 -> tap6/4
  tap5/4 -> tap6/5
  tap5/5 -> tap6/6
  tap5/6 -> tap6/7
  tap5/7 -> tap6/8
  tap5/8 -> tap6/9
  tap5/9 -> tap6/10
  tap6/1 -> tap7/2
  tap6/2 -> tap7/3
  tap6/3 -> tap7/4
  tap6/4 -> tap7/5
  tap6/5 -> tap7/6
  tap6/6 -> tap7/7
  tap6/7 -> tap7/8
  tap6/8 -> tap7/9
  tap6/9 -> tap7/10
  tap7/1 -> tap8/2
  tap7/2 -> tap8/3
  tap7/3 -> tap8/4
  tap7/4 -> tap8/5
  tap7/5 -> tap8/6
  tap7/6 -> tap8/7
  tap7/7 -> tap8/8
  tap7/8 -> tap8/9
  tap7/9 -> tap8/10
  tap8/1 -> tap9/2
  tap8/2 -> tap9/3
  tap8/3 -> tap9/4
  tap8/4 -> tap9/5
  tap8/5 -> tap9/6
  tap8/6 -> tap9/7
  tap8/7 -> tap9/8
  tap8/8 -> tap9/9
  tap8/9 -> tap9/10
  tap9/1 -> tap10/2
  tap9/2 -> tap10/3
  tap9/3 -> tap10/4
  tap9/4 -> tap10/5
  tap9/5 -> tap10/6
  tap9/6 -> tap10/7
  tap9/7 -> tap10/8
  tap9/8 -> tap10/9
  tap9/9 -> tap10/10
  tap10/1 -> tap11/2
  tap10/2 -> tap11/3
  tap10/3 -> tap11/4
  tap10/4 -> tap11/5
  tap10/5 -> tap11/6
  tap10/6 -> tap11/7
  tap10/7 -> tap11/8
  tap10/8 -> tap11/9
  tap10/9 -> tap11/10
  tap11/1 -> tap12/2
  tap11/2 -> tap12/3
  tap11/3 -> tap12/4
  tap11/4 -> tap12/5
  tap11/5 -> tap12/6
  tap11/6 -> tap12/7
  tap11/7 -> tap12/8
  tap11/8 -> tap12/9
  tap11/9 -> tap12/10
  tap12/1 -> tap13/2
  tap12/2 -> tap13/3
  tap12/3 -> tap13/4
  tap12/4 -> tap13/5
  tap12/5 -> tap13/6
  tap12/6 -> tap13/7
  tap12/7 -> tap13/8
  tap12/8 -> tap13/9
  tap12/9 -> tap13/10
  tap13/1 -> tap14/2
  tap13/2 -> tap14/3
  tap13/3 -> tap14/4
  tap13/4 -> tap14/5
  tap13/5 -> tap14/6
  tap13/6 -> tap14/7
  tap13/7 -> tap14/8
  tap13/8 -> tap14/9
  tap13/9 -> tap14/10
  tap14/1 -> tap15/2
  tap14/2 -> tap15/3
  tap14/3 -> tap15/4
  tap14/4 -> tap15/5
  tap14/5 -> tap15/6
  tap14/6 -> tap15/7
  tap14/7 -> tap15/8
  tap14/8 -> tap15/9
  tap14/9 -> tap15/10
  tap15/1 -> tap16/2
  tap15/2 -> tap16/3
  tap15/3 -> tap16/4
  tap15/4 -> tap16/5
  tap15/5 -> tap16/6
  tap15/6 -> tap16/7
  tap15/7 -> tap16/8
  tap15/8 -> tap16/9
  tap15/9 -> tap16/10
  tap16/1 -> tap17/2
  tap16/2 -> tap17/3
  tap16/3 -> tap17/4
  tap16/4 -> tap17/5
  tap16/5 -> tap17/6
  tap16/6 -> tap17/7
  tap16/7 -> tap17/8
  tap16/8 -> tap17/9
  tap16/9 -> tap17/10
  tap17/1 -> tap18/2
  tap17/2 -> tap18/3
  tap17/3 -> tap18/4
  tap17/4 -> tap18/5
  tap17/5 -> tap18/6
  tap17/6 -> tap18/7
  tap17/7 -> tap18/8
  tap17/8 -> tap18/9
  tap17/9 -> tap18/10
  tap18/1 -> tap19/2
  tap18/2 -> tap19/3
  tap18/3 -> tap19/4
  tap18/4 -> tap19/5
  tap18/5 -> tap19/6
  tap18/6 -> tap19/7
  tap18/7 -> tap19/8
  tap18/8 -> tap19/9
  tap18/9 -> tap19/10
  tap19/1 -> tap20/2
  tap19/2 -> tap20/3
  tap19/3 -> tap20/4
  tap19/4 -> tap20/5
  tap19/5 -> tap20/6
  tap19/6 -> tap20/7
  tap19/7 -> tap20/8
  tap19/8 -> tap20/9
  tap19/9 -> tap20/10
  tap20/10 -> fil_out_1/1
  tap20/11 -> fil_out_2/1
  tap20/12 -> fil_out_3/1
  tap20/13 -> fil_out_4/1

== system beamform/Subsystem ==
  set : Inport  OutDataType=sfix(16)  OutScaling=2^0
  reset : Inport  Port=2  OutDataType=sfix(16)  OutScaling=2^0
  Constant1 : xbsIndex_r4/Constant  arith_type=Unsigned  const=1  n_bits=1  bin_pt=0  explicit_period=off  period=1  equ=P=C  opselect=C  inp2=PCIN>>17  opr=+  inp1=P  carry=CIN  dbl_ovrd=off  block_type=constant
  Mux : xbsIndex_r4/Mux  inputs=2  en=off  latency=0  precision=Full  arith_type="Signed  (2's comp)"  n_bits=8  bin_pt=2  quantization=Truncate  overflow=Wrap  dbl_ovrd=off  block_type=mux
      settings: xl_area=[0, 0, 0, 0, 0, 0, 0]
  Register : xbsIndex_r4/Register  init=0  rst=on  en=off  dbl_ovrd=off  block_type=register
      settings: xl_area=[0, 0, 0, 0, 0, 0, 0]
  out : Outport  OutDataType=sfix(16)  OutScaling=2^0
  wires:
  Constant1/1 -> Mux/3
  Mux/1 -> Register/1
  Register/1 -> Mux/2, out/1
  set/1 -> Mux/1
  reset/1 -> Register/2

== system beamform/demux ==
  sel : Inport  OutDataType=sfix(16)  OutScaling=2^0
  In : Inport  Port=2  OutDataType=sfix(16)  OutScaling=2^0
  Subsystem : Subsystem
  Subsystem1 : Subsystem
  Subsystem2 : Subsystem
  Subsystem3 : Subsystem
  Out1 : Outport  OutDataType=sfix(16)  OutScaling=2^0
  Out2 : Outport  Port=2  OutDataType=sfix(16)  OutScaling=2^0
  Out3 : Outport  Port=3  OutDataType=sfix(16)  OutScaling=2^0
  Out4 : Outport  Port=4  OutDataType=sfix(16)  OutScaling=2^0
  wires:
  sel/1 -> Subsystem2/1(sel), Subsystem3/1(sel), Subsystem1/1(sel), Subsystem/1(sel)
  Subsystem2/1(out) -> Out1/1
  In/1 -> Subsystem2/2(in0), Subsystem3/2(in1), Subsystem1/2(in2), Subsystem/2(in3)
  Subsystem3/1(out) -> Out2/1
  Subsystem1/1(out) -> Out3/1
  Subsystem/1(out) -> Out4/1

== system beamform/fifodelay ==
  In1 : Inport  OutDataType=sfix(16)  OutScaling=2^0
  In2 : Inport  Port=2  OutDataType=sfix(16)  OutScaling=2^0
  In3 : Inport  Port=3  OutDataType=sfix(16)  OutScaling=2^0
  In4 : Inport  Port=4  OutDataType=sfix(16)  OutScaling=2^0
  Out1 : Outport  OutDataType=sfix(16)  OutScaling=2^0
  Out2 : Outport  Port=2  OutDataType=sfix(16)  OutScaling=2^0

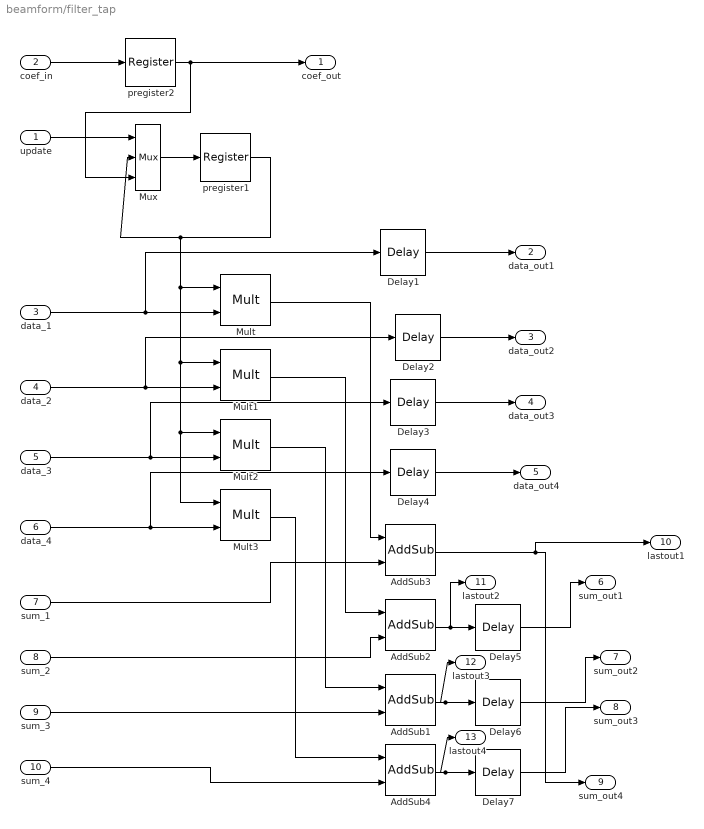
== system beamform/filter_tap ==
  update : Inport  OutDataType=sfix(16)  OutScaling=2^0
  coef_in : Inport  Port=2  OutDataType=sfix(16)  OutScaling=2^0
  data_1 : Inport  Port=3  OutDataType=sfix(16)  OutScaling=2^0
  data_2 : Inport  Port=4  OutDataType=sfix(16)  OutScaling=2^0
  data_3 : Inport  Port=5  OutDataType=sfix(16)  OutScaling=2^0
  data_4 : Inport  Port=6  OutDataType=sfix(16)  OutScaling=2^0
  sum_1 : Inport  Port=7  OutDataType=sfix(16)  OutScaling=2^0
  sum_2 : Inport  Port=8  OutDataType=sfix(16)  OutScaling=2^0
  sum_3 : Inport  Port=9  OutDataType=sfix(16)  OutScaling=2^0
  sum_4 : Inport  Port=10  OutDataType=sfix(16)  OutScaling=2^0
  AddSub{1..4} (4 alike) : xbsIndex_r4/AddSub  mode=Addition  use_carryin=off  use_carryout=off  en=off  latency=add_latency  precision=User Defined  arith_type="Signed  (2's comp)"  n_bits=qn_bits  bin_pt=qbnpnt  quantization=Truncate  overflow=Wrap  dbl_ovrd=off  use_behavioral_HDL=on  pipelined=off  use_rpm=on  hw_selection=Fabric  block_type=addsub
      settings: xl_area=[0, 0, 0, 0, 0, 0, 0]  block_version=10.1.3
  Delay{1..4} (4 alike) : xbsIndex_r4/Delay  en=off  latency=add_latency+1  dbl_ovrd=off  reg_retiming=on  block_type=delay
      settings: xl_area=[0, 0, 0, 0, 0, 0, 0]
  Delay5 : xbsIndex_r4/Delay  en=off  latency=1  dbl_ovrd=off  reg_retiming=on  block_type=delay
      settings: xl_area=[0, 0, 0, 0, 0, 0, 0]
  Delay6 : xbsIndex_r4/Delay  en=off  latency=1  dbl_ovrd=off  reg_retiming=on  block_type=delay
      settings: xl_area=[0, 0, 0, 0, 0, 0, 0]
  Delay7 : xbsIndex_r4/Delay  en=off  latency=1  dbl_ovrd=off  reg_retiming=on  block_type=delay
      settings: xl_area=[0, 0, 0, 0, 0, 0, 0]
  Mult{,1..3} (4 alike) : xbsIndex_r4/Mult  precision=User Defined  arith_type="Signed  (2's comp)"  n_bits=n_bits  bin_pt=bnpnt  quantization=Truncate  overflow=Wrap  en=off  latency=mult_latency  dbl_ovrd=off  use_behavioral_HDL=off  use_embedded=on  opt=Speed  optimum_pipeline=off  pipeline=on  use_rpm=on  placement_style=Rectangular shape  block_type=mult
      settings: infoedit=Hardware notes: To use the internal pipeline stage of the dedicated multiplier you must select 'Pipeline for maximum performance'.  xl_area=[0, 0, 0, 0, 0, 0, 0]  block_version=10.1.3
  Mux : xbsIndex_r4/Mux  inputs=2  en=off  latency=mux_latency  precision=User Defined  arith_type="Signed  (2's comp)"  n_bits=n_bits  bin_pt=bnpnt  quantization=Truncate  overflow=Wrap  dbl_ovrd=off  block_type=mux
      settings: xl_area=[0, 0, 0, 0, 0, 0, 0]
  pregister1 : xbsIndex_r4/Register  init=0  rst=off  en=off  dbl_ovrd=off  block_type=register
      settings: xl_area=[0, 0, 0, 0, 0, 0, 0]
  pregister2 : xbsIndex_r4/Register  init=0  rst=off  en=off  dbl_ovrd=off  block_type=register
      settings: xl_area=[0, 0, 0, 0, 0, 0, 0]
  coef_out : Outport  OutDataType=sfix(16)  OutScaling=2^0
  data_out1 : Outport  Port=2  OutDataType=sfix(16)  OutScaling=2^0
  data_out2 : Outport  Port=3  OutDataType=sfix(16)  OutScaling=2^0
  data_out3 : Outport  Port=4  OutDataType=sfix(16)  OutScaling=2^0
  data_out4 : Outport  Port=5  OutDataType=sfix(16)  OutScaling=2^0
  sum_out1 : Outport  Port=6  OutDataType=sfix(16)  OutScaling=2^0
  sum_out2 : Outport  Port=7  OutDataType=sfix(16)  OutScaling=2^0
  sum_out3 : Outport  Port=8  OutDataType=sfix(16)  OutScaling=2^0
  sum_out4 : Outport  Port=9  OutDataType=sfix(16)  OutScaling=2^0
  lastout1 : Outport  Port=10  OutDataType=sfix(16)  OutScaling=2^0
  lastout2 : Outport  Port=11  OutDataType=sfix(16)  OutScaling=2^0
  lastout3 : Outport  Port=12  OutDataType=sfix(16)  OutScaling=2^0
  lastout4 : Outport  Port=13  OutDataType=sfix(16)  OutScaling=2^0
  wires:
  Mux/1 -> pregister1/1
  pregister1/1 -> Mux/2, Mult/1, Mult2/1, Mult3/1, Mult1/1
  update/1 -> Mux/1
  coef_in/1 -> pregister2/1
  pregister2/1 -> coef_out/1, Mux/3
  data_1/1 -> Mult/2, Delay1/1
  data_2/1 -> Mult1/2, Delay2/1
  data_3/1 -> Mult2/2, Delay3/1
  data_4/1 -> Mult3/2, Delay4/1
  Mult2/1 -> AddSub1/1
  Mult1/1 -> AddSub2/1
  Mult/1 -> AddSub3/1
  Mult3/1 -> AddSub4/1
  Delay1/1 -> data_out1/1
  Delay2/1 -> data_out2/1
  Delay3/1 -> data_out3/1
  Delay4/1 -> data_out4/1
  sum_1/1 -> AddSub3/2
  sum_2/1 -> AddSub2/2
  sum_3/1 -> AddSub1/2
  sum_4/1 -> AddSub4/2
  AddSub3/1 -> lastout1/1, sum_out4/1
  AddSub2/1 -> Delay5/1, lastout2/1
  AddSub1/1 -> Delay6/1, lastout3/1
  AddSub4/1 -> Delay7/1, lastout4/1
  Delay5/1 -> sum_out1/1
  Delay6/1 -> sum_out2/1
  Delay7/1 -> sum_out3/1

== system beamform/neg edge ==
  signal : Inport  OutDataType=sfix(16)  OutScaling=2^0
  Inverter2 : xbsIndex_r4/Inverter  en=off  latency=0  dbl_ovrd=off  block_type=inv
      settings: xl_area=[0, 0, 0, 0, 0, 0, 0]
  Logical1 : xbsIndex_r4/Logical  logical_function=AND  inputs=2  en=off  latency=add_latency  precision=Full  arith_type=Unsigned  n_bits=8  bin_pt=2  align_bp=on  dbl_ovrd=off  block_type=logical
      settings: xl_area=[0, 0, 0, 0, 0, 0, 0]
  pre_load_sent1 : xbsIndex_r4/Register  init=0  rst=off  en=off  dbl_ovrd=off  block_type=register
      settings: xl_area=[0, 0, 0, 0, 0, 0, 0]
  neg_edge : Outport  OutDataType=sfix(16)  OutScaling=2^0
  wires:
  Logical1/1 -> neg_edge/1
  pre_load_sent1/1 -> Logical1/1
  signal/1 -> pre_load_sent1/1, Inverter2/1
  Inverter2/1 -> Logical1/2

== system beamform/pos edge ==
  signal : Inport  OutDataType=sfix(16)  OutScaling=2^0
  Inverter2 : xbsIndex_r4/Inverter  en=off  latency=0  dbl_ovrd=off  block_type=inv
      settings: xl_area=[0, 0, 0, 0, 0, 0, 0]
  Logical1 : xbsIndex_r4/Logical  logical_function=AND  inputs=2  en=off  latency=add_latency  precision=Full  arith_type=Unsigned  n_bits=8  bin_pt=2  align_bp=on  dbl_ovrd=off  block_type=logical
      settings: xl_area=[0, 0, 0, 0, 0, 0, 0]
  pre_load_sent1 : xbsIndex_r4/Register  init=0  rst=off  en=off  dbl_ovrd=off  block_type=register
      settings: xl_area=[0, 0, 0, 0, 0, 0, 0]
  pos_edge : Outport  OutDataType=sfix(16)  OutScaling=2^0
  wires:
  signal/1 -> pre_load_sent1/1, Logical1/2
  pre_load_sent1/1 -> Inverter2/1
  Inverter2/1 -> Logical1/1
  Logical1/1 -> pos_edge/1

== system beamform/Delay Line/FIR filter ==
  pre_load : Inport  OutDataType=sfix(16)  OutScaling=2^0
  data_1 : Inport  Port=2  OutDataType=sfix(16)  OutScaling=2^0
  data_2 : Inport  Port=3  OutDataType=sfix(16)  OutScaling=2^0
  data_3 : Inport  Port=4  OutDataType=sfix(16)  OutScaling=2^0
  data_4 : Inport  Port=5  OutDataType=sfix(16)  OutScaling=2^0
  fdelay : Inport  Port=6  OutDataType=sfix(16)  OutScaling=2^0
  Coeff Pre-Load : beamform/Coeff Pre-Load  SystemSampleTime=-1  N=20  T=10  bin_pnt=6  file='cfile.mat'
      link override Constant: equ=P=C
      link override Constant1: equ=P=C
      link override Constant2: equ=P=C
  Coeff_load : Subsystem  AncestorBlock=beamform/Coeff_load  mask{nfilters=10, ntaps=20}
      mask prompts: nfilters "Number of FD filters"; ntaps "Number of Taps per filter"
      mask init:
      | coef_load;
  Constant : xbsIndex_r4/Constant  arith_type=Unsigned  const=0  n_bits=8  bin_pt=0  explicit_period=off  period=1  equ=P=C  opselect=C  inp2=PCIN>>17  opr=+  inp1=P  carry=CIN  dbl_ovrd=off  block_type=constant
  Dual Port RAM : xbsIndex_r4/Dual Port RAM  depth=20*10  initVector=sin(pi*(0:15)/16)  distributed_mem=Block RAM  init_a=0  init_b=0  rst_a=off  rst_b=off  en_a=off  en_b=off  latency=1  write_mode_A=Read After Write  write_mode_B=Read After Write  dbl_ovrd=off  optimize=Area  use_rpm=off  block_type=dpram
      settings: xl_area=[0, 0, 0, 0, 0, 0, 0]  block_version=10.1.3
  Reinterpret : xbsIndex_r4/Reinterpret  force_arith_type=on  arith_type="Signed  (2's comp)"  force_bin_pt=on  bin_pt=6  block_type=reinterpret
      settings: infoedit="Changes signal type without altering the binary representation.   You can changed the signal between signed and unsigned, and relocate the binary point.<P><P>Hardware notes: In hardware this block costs nothing.<P><P>Example:  Suppose the input is 6 bits wide, signed, with 2 fractional bits, and the output is forced to unsigned with 0 fractional bits.  Then an input of -2.0 (1110.00 in binary 2's complement) becomes an output of 56 (111000 in binary)."  block_version=10.1.3
  Shift Reg : Subsystem  AncestorBlock=beamform/Shift Reg  mask{n=20, bin_point=6}
      mask prompts: n "No of taps"; bin_point "Binary Point"
      mask init:
      | shift_reg;
  Slice : xbsIndex_r4/Slice  nbits=1  boolean_output=on  mode=Lower Bit Location + Width  bit1=0  base1=MSB of Input  bit0=0  base0=LSB of Input  dbl_ovrd=off  block_type=slice
      settings: infoedit="Extracts a given range of bits from each input sample and presents it at the output.  The output type is ordinarily unsigned with binary point at zero, but can be Boolean when the slice is one bit wide.<P><P>Hardware notes: In hardware this block costs nothing."  block_version=10.1.3
  Terminator : Terminator
  neg edge : Subsystem
  neg edge1 : Subsystem
  pos edge : beamform/pos edge  SystemSampleTime=-1  add_latency=1
  fil_1 : Outport  OutDataType=sfix(16)  OutScaling=2^0
  fil_2 : Outport  Port=2  OutDataType=sfix(16)  OutScaling=2^0
  fil_3 : Outport  Port=3  OutDataType=sfix(16)  OutScaling=2^0
  fil_4 : Outport  Port=4  OutDataType=sfix(16)  OutScaling=2^0
  wires:
  Reinterpret/1 -> Shift Reg/2(Serial In)
  neg edge1/1(pos_edge) -> Shift Reg/1(Update)
  neg edge/1(pos_edge) -> Coeff_load/1(load)
  pos edge/1 -> Coeff Pre-Load/1
  Coeff_load/1(load_address) -> Dual Port RAM/4
  Slice/1 -> Dual Port RAM/6
  Coeff Pre-Load/1 -> Dual Port RAM/1
  Coeff Pre-Load/2 -> Dual Port RAM/2
  Dual Port RAM/2 -> Reinterpret/1
  Dual Port RAM/1 -> Terminator/1
  Shift Reg/4(fil_out_4) -> fil_4/1
  Shift Reg/3(fil_out_3) -> fil_3/1
  Shift Reg/2(fil_out_2) -> fil_2/1
  Shift Reg/1(fil_out_1) -> fil_1/1
  data_4/1 -> Shift Reg/6(data_4)
  data_3/1 -> Shift Reg/5(data_3)
  data_2/1 -> Shift Reg/4(data_2)
  data_1/1 -> Shift Reg/3(data_1)
  Coeff Pre-Load/3 -> neg edge/1(signal), Dual Port RAM/3
  Constant/1 -> Dual Port RAM/5, Slice/1
  pre_load/1 -> pos edge/1
  Coeff_load/2(load_on) -> neg edge1/1(signal)
  fdelay/1 -> Coeff_load/2(fdelay)

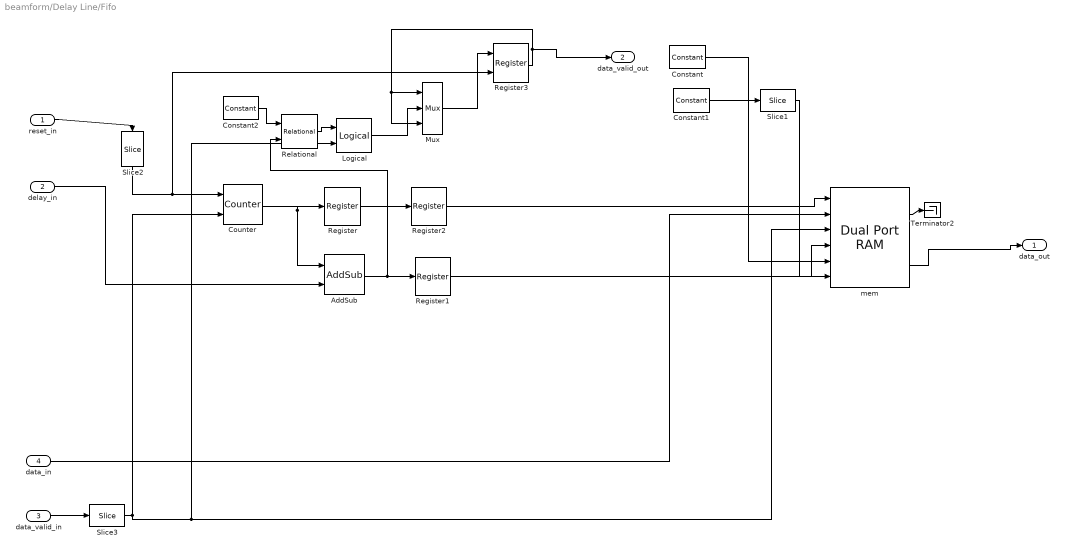
== system beamform/Delay Line/Fifo ==
  reset_in : Inport  OutDataType=sfix(16)  OutScaling=2^0
  delay_in : Inport  Port=2  OutDataType=sfix(16)  OutScaling=2^0
  data_valid_in : Inport  Port=3  OutDataType=sfix(16)  OutScaling=2^0
  data_in : Inport  Port=4  OutDataType=sfix(16)  OutScaling=2^0
  AddSub : xbsIndex_r4/AddSub  mode=Subtraction  use_carryin=off  use_carryout=off  en=off  latency=1  precision=User Defined  arith_type=Unsigned  n_bits=10  bin_pt=0  quantization=Truncate  overflow=Wrap  dbl_ovrd=off  use_behavioral_HDL=on  pipelined=off  use_rpm=on  hw_selection=Fabric  block_type=addsub
      settings: xl_area=[0, 0, 0, 0, 0, 0, 0]  block_version=10.1.3
  Constant : xbsIndex_r4/Constant  arith_type=Unsigned  const=0  n_bits=32  bin_pt=0  explicit_period=on  period=1  equ=P=C  opselect=C  inp2=PCIN>>17  opr=+  inp1=P  carry=CIN  dbl_ovrd=off  block_type=constant
  Constant1 : xbsIndex_r4/Constant  arith_type=Unsigned  const=0  n_bits=1  bin_pt=0  explicit_period=on  period=1  equ=P=C  opselect=C  inp2=PCIN>>17  opr=+  inp1=P  carry=CIN  dbl_ovrd=off  block_type=constant
  Constant2 : xbsIndex_r4/Constant  arith_type=Unsigned  const=0  n_bits=10  bin_pt=0  explicit_period=on  period=1  equ=P=C  opselect=C  inp2=PCIN>>17  opr=+  inp1=P  carry=CIN  dbl_ovrd=off  block_type=constant
  Counter : xbsIndex_r4/Counter  cnt_type=Free Running  cnt_to=Inf  operation=Up  start_count=0  cnt_by_val=1  arith_type=Unsigned  n_bits=10  bin_pt=0  load_pin=off  rst=on  en=on  explicit_period=off  period=1  dbl_ovrd=off  use_behavioral_HDL=off  use_rpm=on  implementation=Fabric  block_type=counter
      settings: xl_area=[0, 0, 0, 0, 0, 0, 0]
  Logical : xbsIndex_r4/Logical  logical_function=AND  inputs=2  en=off  latency=0  precision=Full  arith_type=Unsigned  n_bits=8  bin_pt=2  align_bp=on  dbl_ovrd=off  block_type=logical
      settings: xl_area=[0, 0, 0, 0, 0, 0, 0]
  Mux : xbsIndex_r4/Mux  inputs=2  en=off  latency=0  precision=Full  arith_type="Signed  (2's comp)"  n_bits=8  bin_pt=2  quantization=Truncate  overflow=Wrap  dbl_ovrd=off  block_type=mux
      settings: xl_area=[0, 0, 0, 0, 0, 0, 0]
  Register : xbsIndex_r4/Register  init=0  rst=off  en=off  dbl_ovrd=off  block_type=register
      settings: xl_area=[0, 0, 0, 0, 0, 0, 0]
  Register1 : xbsIndex_r4/Register  init=0  rst=off  en=off  dbl_ovrd=off  block_type=register
      settings: xl_area=[0, 0, 0, 0, 0, 0, 0]
  Register2 : xbsIndex_r4/Register  init=0  rst=off  en=off  dbl_ovrd=off  block_type=register
      settings: xl_area=[0, 0, 0, 0, 0, 0, 0]
  Register3 : xbsIndex_r4/Register  init=0  rst=on  en=off  dbl_ovrd=off  block_type=register
      settings: xl_area=[0, 0, 0, 0, 0, 0, 0]
  Relational : xbsIndex_r4/Relational  mode=a=b  en=off  latency=1  dbl_ovrd=off  block_type=relational
      settings: xl_area=[0, 0, 0, 0, 0, 0, 0]  block_version=10.1.3
  Slice1 : xbsIndex_r4/Slice  nbits=1  boolean_output=on  mode=Upper Bit Location + Width  bit1=0  base1=LSB of Input  bit0=0  base0=LSB of Input  dbl_ovrd=off  block_type=slice
      settings: infoedit="Extracts a given range of bits from each input sample and presents it at the output.  The output type is ordinarily unsigned with binary point at zero, but can be Boolean when the slice is one bit wide.<P><P>Hardware notes: In hardware this block costs nothing."  block_version=10.1.3
  Slice2 : xbsIndex_r4/Slice  Orientation=down  nbits=1  boolean_output=on  mode=Upper Bit Location + Width  bit1=0  base1=LSB of Input  bit0=0  base0=LSB of Input  dbl_ovrd=off  block_type=slice
      settings: infoedit="Extracts a given range of bits from each input sample and presents it at the output.  The output type is ordinarily unsigned with binary point at zero, but can be Boolean when the slice is one bit wide.<P><P>Hardware notes: In hardware this block costs nothing."  block_version=10.1.3
  Slice3 : xbsIndex_r4/Slice  nbits=1  boolean_output=on  mode=Upper Bit Location + Width  bit1=0  base1=LSB of Input  bit0=0  base0=LSB of Input  dbl_ovrd=off  block_type=slice
      settings: infoedit="Extracts a given range of bits from each input sample and presents it at the output.  The output type is ordinarily unsigned with binary point at zero, but can be Boolean when the slice is one bit wide.<P><P>Hardware notes: In hardware this block costs nothing."  block_version=10.1.3
  Terminator2 : Terminator
  mem : xbsIndex_r4/Dual Port RAM  depth=2048  initVector=zeros(1,2048)  distributed_mem=Block RAM  init_a=0  init_b=0  rst_a=off  rst_b=off  en_a=off  en_b=off  latency=1  write_mode_A=Read Before Write  write_mode_B=No Read On Write  dbl_ovrd=off  optimize=Speed  use_rpm=on  block_type=dpram
      settings: block_version=10.1.3
  data_out : Outport  OutDataType=sfix(16)  OutScaling=2^0
  data_valid_out : Outport  Port=2  OutDataType=sfix(16)  OutScaling=2^0
  wires:
  mem/2 -> data_out/1
  mem/1 -> Terminator2/1
  Constant/1 -> mem/5
  Constant1/1 -> Slice1/1
  Slice1/1 -> mem/6
  reset_in/1 -> Slice2/1
  data_valid_in/1 -> Slice3/1
  Counter/1 -> AddSub/1, Register/1
  delay_in/1 -> AddSub/2
  AddSub/1 -> Register1/1, Relational/2
  Register/1 -> Register2/1
  Register2/1 -> mem/1
  Register1/1 -> mem/4
  data_in/1 -> mem/2
  Slice3/1 -> Counter/2, Logical/2, mem/3
  Slice2/1 -> Counter/1, Register3/2
  Mux/1 -> Register3/1
  Register3/1 -> Mux/1, Mux/3, data_valid_out/1
  Constant2/1 -> Relational/1
  Relational/1 -> Logical/1
  Logical/1 -> Mux/2
